simulink model "ctrl_TAPM_2016"  (R2016a)
settings: Solver=ode3  StartTime=0.0  StopTime=inf  FixedStep=0.01  RelTol=1e-3
undefined symbols (not defined in the file): C, D, DiscIntNeverNeededParam, eps_c, epsilon, hd, hd2, I_s, k_cc, K_omega, K_q1f, K_q1r, K_q2f, K_q2r, K_q3f, K_q3r, K_q4f, K_q4r, K_q5f, K_q5r, K_q6f, K_q6r, K_T1f, K_T1r, K_T2f, K_T2r, K_T3f, K_T3r, K_T4f, K_T4r, K_T5f, K_T5r, K_T6f, K_T6r, Kp, Max_Acceleration, Max_rotation, Max_thrust, Min_thrust, n_c, n_max, p_cc, pwm_thr1_backward, pwm_thr1_forward, pwm_thr2_backward, pwm_thr2_forward, pwm_thr3_backward, pwm_thr3_forward, pwm_thr4_backward, pwm_thr4_forward, pwm_thr5_backward, pwm_thr5_forward, pwm_thr6_backward, pwm_thr6_forward, Q_f0, Q_max, r_cc, Rho, Thruster
libraries: marine_gnc x10, dspstat3 x8, simulink x7, simulink_extras x3
(part 4 of 7)

== system ctrl_TAPM_2016/Thruster control  ==
  "Desired thrust and angle " : Inport
  Delay : Delay  DelayLength=1  InitialCondition=0
  Demux : Demux  Outputs=12
  Mapping shaft speed and thrust : Selector  InputPortWidth=12  IndexOptions=Index vector (dialog)  Indices="[1 7 2  8 3 9 4 10 5 11 6 12]"  OutputSizes=1
  Mux : Mux  Inputs=12
  Mux1 : Mux  Inputs=2
  Selecting Desired thrust1 : Selector  InputPortWidth=12  IndexOptions=Index vector (dialog)  Indices=[7 8 9 10 11 12]  OutputSizes=1
  Selecting actual angle : Selector  InputPortWidth=12  IndexOptions=Index vector (dialog)  Indices=[1 2 3 4 5 6]  OutputSizes=1
  Subsystem1 : Subsystem
  Thrust and Shaft speed mapped to PWM : Subsystem
  Thruster 1 : Subsystem
      settings: AttributesFormatString=%<MinAlgLoopOccurrences>
  Thruster 2 : Subsystem
      settings: AttributesFormatString=%<MinAlgLoopOccurrences>
  Thruster 3 : Subsystem
      settings: AttributesFormatString=%<MinAlgLoopOccurrences>
  Thruster 4 : Subsystem
      settings: AttributesFormatString=%<MinAlgLoopOccurrences>
  Thruster 5 : Subsystem
      settings: AttributesFormatString=%<MinAlgLoopOccurrences>
  Thruster 6 : Subsystem
      settings: AttributesFormatString=%<MinAlgLoopOccurrences>
  "Commanded pwm " : Outport
  Commanded angle : Outport  Port=2
  Commanded thrust : Outport  Port=3
  wires:
  Selecting actual angle/1 -> Subsystem1/1(Calculated angles)
  "Desired thrust and angle "/1 -> Selecting actual angle/1, Selecting Desired thrust1/1
  Subsystem1/1(Commanded angles) -> Commanded angle/1
  Thrust and Shaft speed mapped to PWM/1(pwm) -> "Commanded pwm "/1
  Thrust and Shaft speed mapped to PWM/2(Force) -> Commanded thrust/1
  Thrust and Shaft speed mapped to PWM/3("Shaft speed ") -> Delay/1
  Thruster 1/1("Commanded thrust ") -> Mux/1
  Mux/1 -> Thrust and Shaft speed mapped to PWM/1(Calculated thrust)
  Mux1/1 -> Mapping shaft speed and thrust/1
  Delay/1 -> Mux1/2
  Mapping shaft speed and thrust/1 -> Demux/1
  Thruster 1/2(Shaft speed) -> Mux/2
  Demux/2 -> Thruster 1/2(shaft speed)
  Demux/1 -> Thruster 1/1(Desired thrust 1)
  Thruster 2/1("Commanded thrust ") -> Mux/3
  Demux/3 -> Thruster 2/1(Desired thrust 1)
  Demux/4 -> Thruster 2/2(shaft speed)
  Demux/5 -> Thruster 3/1(Desired thrust 1)
  Demux/6 -> Thruster 3/2(shaft speed)
  Demux/7 -> Thruster 4/1(Desired thrust 1)
  Demux/8 -> Thruster 4/2(shaft speed)
  Demux/9 -> Thruster 5/1(Desired thrust 1)
  Demux/10 -> Thruster 5/2(shaft speed)
  Demux/11 -> Thruster 6/1(Desired thrust 1)
  Demux/12 -> Thruster 6/2(shaft speed)
  Thruster 2/2(Shaft speed) -> Mux/4
  Thruster 3/1("Commanded thrust ") -> Mux/5
  Thruster 3/2(Shaft speed) -> Mux/6
  Thruster 4/1("Commanded thrust ") -> Mux/7
  Thruster 4/2(Shaft speed) -> Mux/8
  Thruster 5/1("Commanded thrust ") -> Mux/9
  Thruster 5/2(Shaft speed) -> Mux/10
  Thruster 6/1("Commanded thrust ") -> Mux/11
  Thruster 6/2(Shaft speed) -> Mux/12
  Selecting Desired thrust1/1 -> Mux1/1

== system ctrl_TAPM_2016/Thruster measurment ==
  Mux1 : Mux  Inputs=6
  thr_angle_1 : S-Function  Priority=1  FunctionName=NIVeriStandIO  Parameters=width dtype portnum stime stype btype  SFunctionDeploymentMode=off  EnableBusSupport=off  mask(NI VeriStand Inport){portnum=1, width=-1, stime=-1, dtype=auto, stype=auto, btype=1}
      mask prompts: portnum "Port number:"; width "Port dimensions (-1 for dynamically sized):"; stime "Sample time (-1 for inherited):"; dtype "Data type:"; stype "Signal type:"; btype "Block type:"
      mask help: Use this inport on any level of nested subsystems to allow NI VeriStand software to map signals to it.
      mask init:
      | NIVeriStandIO_init;
      settings: CopyFcn=NIVeriStand_MDL_functions('', 'IO_copy');  DeleteFcn=NIVeriStand_MDL_functions('', 'IO_delete');  MoveFcn=set_param(gcb, 'Mask', 'on');
      mask Callback portnum: NIVeriStand_MDL_functions('', 'IO_setportnum');
      mask TypeOptions dtype: auto | double | single | int8 | uint8 | int16 | uint16 | int32 | uint32 | boolean
      mask Callback dtype: NIVeriStand_MDL_functions('', 'IO_booleansignal');
      mask TypeOptions stype: auto | real | complex
      mask Display:
      | patch([-x x], [-y y], [.90980 .81960 .32156]);
      | plot([xrad -x x xrad], [yrad -y y yrad]);
      | fprintf('NI In%d', portnum);
  thr_angle_2 : S-Function  Priority=2  FunctionName=NIVeriStandIO  Parameters=width dtype portnum stime stype btype  SFunctionDeploymentMode=off  EnableBusSupport=off  mask(NI VeriStand Inport){portnum=2, width=-1, stime=-1, dtype=auto, stype=auto, btype=1}
      mask prompts: portnum "Port number:"; width "Port dimensions (-1 for dynamically sized):"; stime "Sample time (-1 for inherited):"; dtype "Data type:"; stype "Signal type:"; btype "Block type:"
      mask help: Use this inport on any level of nested subsystems to allow NI VeriStand software to map signals to it.
      mask init:
      | NIVeriStandIO_init;
      settings: CopyFcn=NIVeriStand_MDL_functions('', 'IO_copy');  DeleteFcn=NIVeriStand_MDL_functions('', 'IO_delete');  MoveFcn=set_param(gcb, 'Mask', 'on');
      mask Callback portnum: NIVeriStand_MDL_functions('', 'IO_setportnum');
      mask TypeOptions dtype: auto | double | single | int8 | uint8 | int16 | uint16 | int32 | uint32 | boolean
      mask Callback dtype: NIVeriStand_MDL_functions('', 'IO_booleansignal');
      mask TypeOptions stype: auto | real | complex
      mask Display:
      | patch([-x x], [-y y], [.90980 .81960 .32156]);
      | plot([xrad -x x xrad], [yrad -y y yrad]);
      | fprintf('NI In%d', portnum);
  thr_angle_3 : S-Function  Priority=3  FunctionName=NIVeriStandIO  Parameters=width dtype portnum stime stype btype  SFunctionDeploymentMode=off  EnableBusSupport=off  mask(NI VeriStand Inport){portnum=3, width=-1, stime=-1, dtype=auto, stype=auto, btype=1}
      mask prompts: portnum "Port number:"; width "Port dimensions (-1 for dynamically sized):"; stime "Sample time (-1 for inherited):"; dtype "Data type:"; stype "Signal type:"; btype "Block type:"
      mask help: Use this inport on any level of nested subsystems to allow NI VeriStand software to map signals to it.
      mask init:
      | NIVeriStandIO_init;
      settings: CopyFcn=NIVeriStand_MDL_functions('', 'IO_copy');  DeleteFcn=NIVeriStand_MDL_functions('', 'IO_delete');  MoveFcn=set_param(gcb, 'Mask', 'on');
      mask Callback portnum: NIVeriStand_MDL_functions('', 'IO_setportnum');
      mask TypeOptions dtype: auto | double | single | int8 | uint8 | int16 | uint16 | int32 | uint32 | boolean
      mask Callback dtype: NIVeriStand_MDL_functions('', 'IO_booleansignal');
      mask TypeOptions stype: auto | real | complex
      mask Display:
      | patch([-x x], [-y y], [.90980 .81960 .32156]);
      | plot([xrad -x x xrad], [yrad -y y yrad]);
      | fprintf('NI In%d', portnum);
  thr_angle_4 : S-Function  Priority=4  FunctionName=NIVeriStandIO  Parameters=width dtype portnum stime stype btype  SFunctionDeploymentMode=off  EnableBusSupport=off  mask(NI VeriStand Inport){portnum=4, width=-1, stime=-1, dtype=auto, stype=auto, btype=1}
      mask prompts: portnum "Port number:"; width "Port dimensions (-1 for dynamically sized):"; stime "Sample time (-1 for inherited):"; dtype "Data type:"; stype "Signal type:"; btype "Block type:"
      mask help: Use this inport on any level of nested subsystems to allow NI VeriStand software to map signals to it.
      mask init:
      | NIVeriStandIO_init;
      settings: CopyFcn=NIVeriStand_MDL_functions('', 'IO_copy');  DeleteFcn=NIVeriStand_MDL_functions('', 'IO_delete');  MoveFcn=set_param(gcb, 'Mask', 'on');
      mask Callback portnum: NIVeriStand_MDL_functions('', 'IO_setportnum');
      mask TypeOptions dtype: auto | double | single | int8 | uint8 | int16 | uint16 | int32 | uint32 | boolean
      mask Callback dtype: NIVeriStand_MDL_functions('', 'IO_booleansignal');
      mask TypeOptions stype: auto | real | complex
      mask Display:
      | patch([-x x], [-y y], [.90980 .81960 .32156]);
      | plot([xrad -x x xrad], [yrad -y y yrad]);
      | fprintf('NI In%d', portnum);
  thr_angle_5 : S-Function  Priority=5  FunctionName=NIVeriStandIO  Parameters=width dtype portnum stime stype btype  SFunctionDeploymentMode=off  EnableBusSupport=off  mask(NI VeriStand Inport){portnum=5, width=-1, stime=-1, dtype=auto, stype=auto, btype=1}
      mask prompts: portnum "Port number:"; width "Port dimensions (-1 for dynamically sized):"; stime "Sample time (-1 for inherited):"; dtype "Data type:"; stype "Signal type:"; btype "Block type:"
      mask help: Use this inport on any level of nested subsystems to allow NI VeriStand software to map signals to it.
      mask init:
      | NIVeriStandIO_init;
      settings: CopyFcn=NIVeriStand_MDL_functions('', 'IO_copy');  DeleteFcn=NIVeriStand_MDL_functions('', 'IO_delete');  MoveFcn=set_param(gcb, 'Mask', 'on');
      mask Callback portnum: NIVeriStand_MDL_functions('', 'IO_setportnum');
      mask TypeOptions dtype: auto | double | single | int8 | uint8 | int16 | uint16 | int32 | uint32 | boolean
      mask Callback dtype: NIVeriStand_MDL_functions('', 'IO_booleansignal');
      mask TypeOptions stype: auto | real | complex
      mask Display:
      | patch([-x x], [-y y], [.90980 .81960 .32156]);
      | plot([xrad -x x xrad], [yrad -y y yrad]);
      | fprintf('NI In%d', portnum);
  thr_angle_6 : S-Function  Priority=6  FunctionName=NIVeriStandIO  Parameters=width dtype portnum stime stype btype  SFunctionDeploymentMode=off  EnableBusSupport=off  mask(NI VeriStand Inport){portnum=6, width=-1, stime=-1, dtype=auto, stype=auto, btype=1}
      mask prompts: portnum "Port number:"; width "Port dimensions (-1 for dynamically sized):"; stime "Sample time (-1 for inherited):"; dtype "Data type:"; stype "Signal type:"; btype "Block type:"
      mask help: Use this inport on any level of nested subsystems to allow NI VeriStand software to map signals to it.
      mask init:
      | NIVeriStandIO_init;
      settings: CopyFcn=NIVeriStand_MDL_functions('', 'IO_copy');  DeleteFcn=NIVeriStand_MDL_functions('', 'IO_delete');  MoveFcn=set_param(gcb, 'Mask', 'on');
      mask Callback portnum: NIVeriStand_MDL_functions('', 'IO_setportnum');
      mask TypeOptions dtype: auto | double | single | int8 | uint8 | int16 | uint16 | int32 | uint32 | boolean
      mask Callback dtype: NIVeriStand_MDL_functions('', 'IO_booleansignal');
      mask TypeOptions stype: auto | real | complex
      mask Display:
      | patch([-x x], [-y y], [.90980 .81960 .32156]);
      | plot([xrad -x x xrad], [yrad -y y yrad]);
      | fprintf('NI In%d', portnum);
  alpha_m : Outport
  wires:
  thr_angle_3/1 -> Mux1/3
  thr_angle_1/1 -> Mux1/1
  Mux1/1 -> alpha_m/1
  thr_angle_5/1 -> Mux1/5
  thr_angle_4/1 -> Mux1/4
  thr_angle_6/1 -> Mux1/6
  thr_angle_2/1 -> Mux1/2

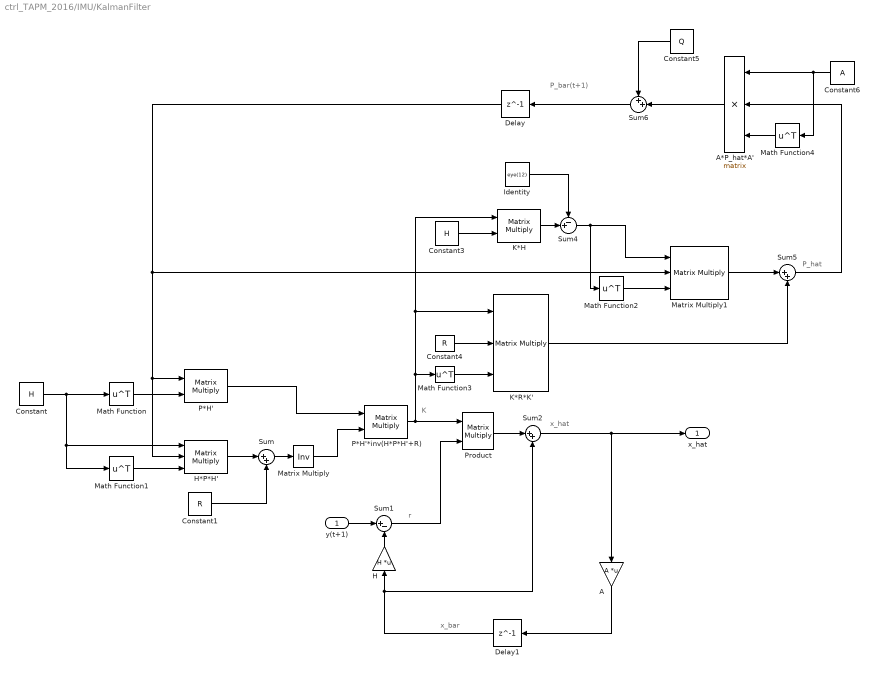
== system ctrl_TAPM_2016/IMU/KalmanFilter ==
  note: P_bar(t+1)
  note: P_hat
  note: x_hat
  note: x_bar
  note: r
  note: K
  y(t+1) : Inport
  A : Gain  Gain=A  Multiplication=Matrix(K*u)
  A*P_hat*A' : Product  Inputs=3  Multiplication=Matrix(*)
  Constant : Constant  Value=H
  Constant1 : Constant  Value=R
  Constant3 : Constant  Value=H
  Constant4 : Constant  Value=R
  Constant5 : Constant  Value=Q
  Constant6 : Constant  Value=A
  Delay : Delay  DelayLength=1  InitialCondition=eye(12)
  Delay1 : Delay  DelayLength=1  InitialCondition=[0 0 0 0 0 0 0 0 0 0 0 0]
  H : Gain  Gain=H  Multiplication=Matrix(K*u)
  H*P*H' : Product  Inputs=3  Multiplication=Matrix(*)
  Identity : Constant  Value=eye(12)
  K*H : Product  Multiplication=Matrix(*)
  K*R*K' : Product  Inputs=3  Multiplication=Matrix(*)
  Math Function{,1..4} (5 alike) : Math  Operator=transpose  SaturateOnIntegerOverflow=on
  Matrix Multiply : Product  Inputs=/  Multiplication=Matrix(*)
  Matrix Multiply1 : Product  Inputs=3  Multiplication=Matrix(*)
  P*H' : Product  Multiplication=Matrix(*)
  P*H'*inv(H*P*H'+R) : Product  Multiplication=Matrix(*)
  Product : Product  Multiplication=Matrix(*)
  Sum : Sum  Inputs=|++
  Sum1 : Sum  Inputs=|+-
  Sum2 : Sum  Inputs=|++
  Sum4 : Sum  Inputs=-+|
  Sum5 : Sum  Inputs=|++
  Sum6 : Sum  Inputs=++|
  x_hat : Outport
  wires:
  Constant/1 -> Math Function1/1, H*P*H'/1, Math Function/1
  Math Function/1 -> P*H'/2
  Math Function1/1 -> H*P*H'/3
  H*P*H'/1 -> Sum/1
  Constant1/1 -> Sum/2
  Sum/1 -> Matrix Multiply/1
  Matrix Multiply/1 -> P*H'*inv(H*P*H'+R)/2
  P*H'/1 -> P*H'*inv(H*P*H'+R)/1
  y(t+1)/1 -> Sum1/1
  H/1 -> Sum1/2
  Delay1/1 -> Sum2/2, H/1
  Sum1/1 -> Product/2
  P*H'*inv(H*P*H'+R)/1 -> K*H/1, K*R*K'/1, Math Function3/1, Product/1
  Product/1 -> Sum2/1
  Sum2/1 -> A/1, x_hat/1
  A/1 -> Delay1/1
  Identity/1 -> Sum4/1
  K*H/1 -> Sum4/2
  Constant3/1 -> K*H/2
  Sum4/1 -> Math Function2/1, Matrix Multiply1/1
  Math Function2/1 -> Matrix Multiply1/3
  Constant4/1 -> K*R*K'/2
  Math Function3/1 -> K*R*K'/3
  K*R*K'/1 -> Sum5/2
  Matrix Multiply1/1 -> Sum5/1
  Sum5/1 -> A*P_hat*A'/2
  Sum6/1 -> Delay/1
  Constant5/1 -> Sum6/1
  A*P_hat*A'/1 -> Sum6/2
  Constant6/1 -> Math Function4/1, A*P_hat*A'/1
  Math Function4/1 -> A*P_hat*A'/3
  Delay/1 -> H*P*H'/2, P*H'/1, Matrix Multiply1/2

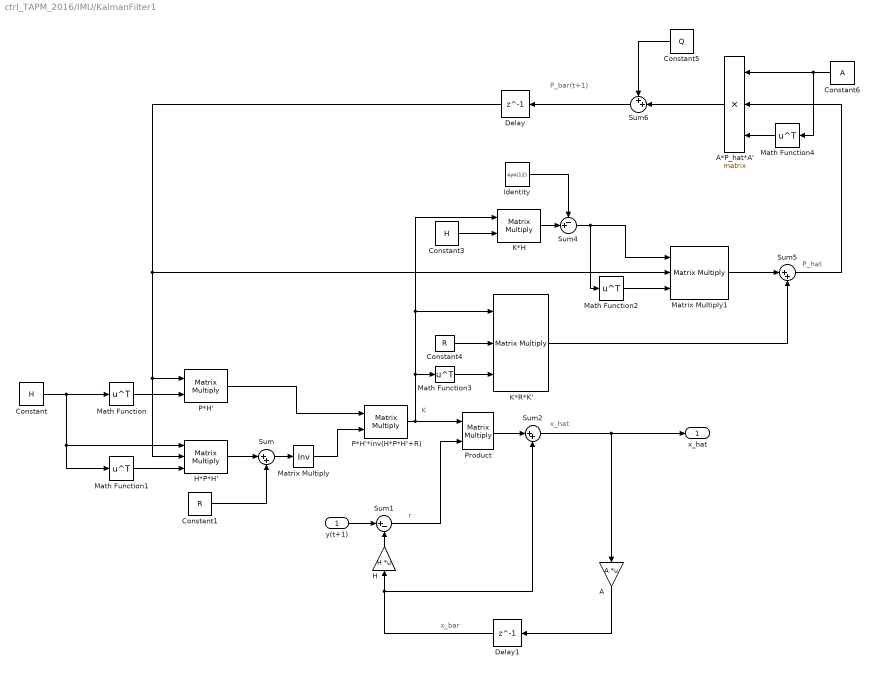
== system ctrl_TAPM_2016/IMU/KalmanFilter1 ==
  note: P_bar(t+1)
  note: P_hat
  note: x_hat
  note: x_bar
  note: r
  note: K
  y(t+1) : Inport
  A : Gain  Gain=A  Multiplication=Matrix(K*u)
  A*P_hat*A' : Product  Inputs=3  Multiplication=Matrix(*)
  Constant : Constant  Value=H
  Constant1 : Constant  Value=R
  Constant3 : Constant  Value=H
  Constant4 : Constant  Value=R
  Constant5 : Constant  Value=Q
  Constant6 : Constant  Value=A
  Delay : Delay  DelayLength=1  InitialCondition=eye(12)
  Delay1 : Delay  DelayLength=1  InitialCondition=[0 0 0 0 0 0 0 0 0 0 0 0]
  H : Gain  Gain=H  Multiplication=Matrix(K*u)
  H*P*H' : Product  Inputs=3  Multiplication=Matrix(*)
  Identity : Constant  Value=eye(12)
  K*H : Product  Multiplication=Matrix(*)
  K*R*K' : Product  Inputs=3  Multiplication=Matrix(*)
  Math Function{,1..4} (5 alike) : Math  Operator=transpose  SaturateOnIntegerOverflow=on
  Matrix Multiply : Product  Inputs=/  Multiplication=Matrix(*)
  Matrix Multiply1 : Product  Inputs=3  Multiplication=Matrix(*)
  P*H' : Product  Multiplication=Matrix(*)
  P*H'*inv(H*P*H'+R) : Product  Multiplication=Matrix(*)
  Product : Product  Multiplication=Matrix(*)
  Sum : Sum  Inputs=|++
  Sum1 : Sum  Inputs=|+-
  Sum2 : Sum  Inputs=|++
  Sum4 : Sum  Inputs=-+|
  Sum5 : Sum  Inputs=|++
  Sum6 : Sum  Inputs=++|
  x_hat : Outport
  wires:
  Constant/1 -> Math Function1/1, H*P*H'/1, Math Function/1
  Math Function/1 -> P*H'/2
  Math Function1/1 -> H*P*H'/3
  H*P*H'/1 -> Sum/1
  Constant1/1 -> Sum/2
  Sum/1 -> Matrix Multiply/1
  Matrix Multiply/1 -> P*H'*inv(H*P*H'+R)/2
  P*H'/1 -> P*H'*inv(H*P*H'+R)/1
  y(t+1)/1 -> Sum1/1
  H/1 -> Sum1/2
  Delay1/1 -> Sum2/2, H/1
  Sum1/1 -> Product/2
  P*H'*inv(H*P*H'+R)/1 -> K*H/1, K*R*K'/1, Math Function3/1, Product/1
  Product/1 -> Sum2/1
  Sum2/1 -> A/1, x_hat/1
  A/1 -> Delay1/1
  Identity/1 -> Sum4/1
  K*H/1 -> Sum4/2
  Constant3/1 -> K*H/2
  Sum4/1 -> Math Function2/1, Matrix Multiply1/1
  Math Function2/1 -> Matrix Multiply1/3
  Constant4/1 -> K*R*K'/2
  Math Function3/1 -> K*R*K'/3
  K*R*K'/1 -> Sum5/2
  Matrix Multiply1/1 -> Sum5/1
  Sum5/1 -> A*P_hat*A'/2
  Sum6/1 -> Delay/1
  Constant5/1 -> Sum6/1
  A*P_hat*A'/1 -> Sum6/2
  Constant6/1 -> Math Function4/1, A*P_hat*A'/1
  Math Function4/1 -> A*P_hat*A'/3
  Delay/1 -> H*P*H'/2, P*H'/1, Matrix Multiply1/2

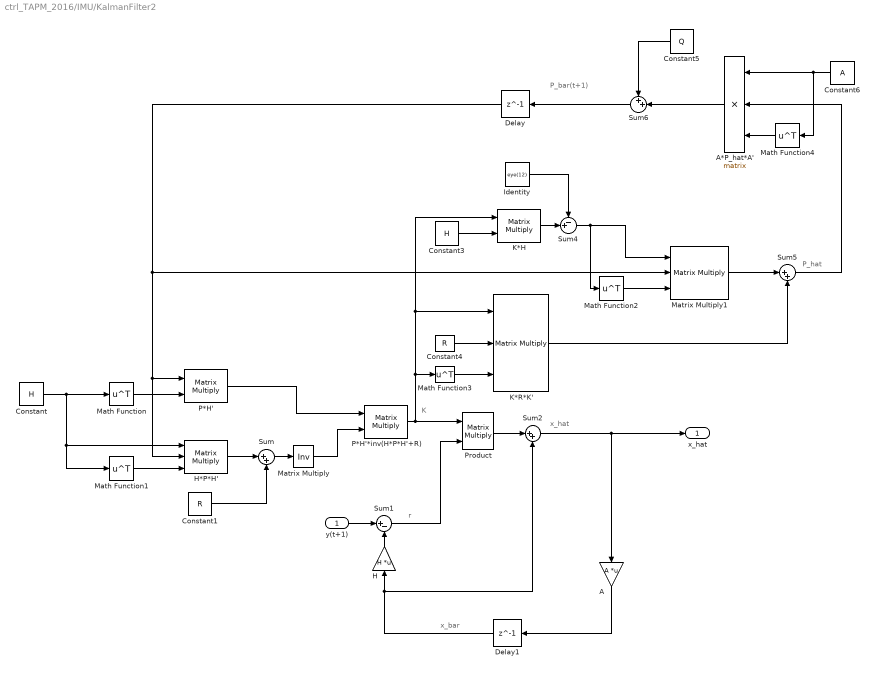
== system ctrl_TAPM_2016/IMU/KalmanFilter2 ==
  note: P_bar(t+1)
  note: P_hat
  note: x_hat
  note: x_bar
  note: r
  note: K
  y(t+1) : Inport
  A : Gain  Gain=A  Multiplication=Matrix(K*u)
  A*P_hat*A' : Product  Inputs=3  Multiplication=Matrix(*)
  Constant : Constant  Value=H
  Constant1 : Constant  Value=R
  Constant3 : Constant  Value=H
  Constant4 : Constant  Value=R
  Constant5 : Constant  Value=Q
  Constant6 : Constant  Value=A
  Delay : Delay  DelayLength=1  InitialCondition=eye(12)
  Delay1 : Delay  DelayLength=1  InitialCondition=[0 0 0 0 0 0 0 0 0 0 0 0]
  H : Gain  Gain=H  Multiplication=Matrix(K*u)
  H*P*H' : Product  Inputs=3  Multiplication=Matrix(*)
  Identity : Constant  Value=eye(12)
  K*H : Product  Multiplication=Matrix(*)
  K*R*K' : Product  Inputs=3  Multiplication=Matrix(*)
  Math Function{,1..4} (5 alike) : Math  Operator=transpose  SaturateOnIntegerOverflow=on
  Matrix Multiply : Product  Inputs=/  Multiplication=Matrix(*)
  Matrix Multiply1 : Product  Inputs=3  Multiplication=Matrix(*)
  P*H' : Product  Multiplication=Matrix(*)
  P*H'*inv(H*P*H'+R) : Product  Multiplication=Matrix(*)
  Product : Product  Multiplication=Matrix(*)
  Sum : Sum  Inputs=|++
  Sum1 : Sum  Inputs=|+-
  Sum2 : Sum  Inputs=|++
  Sum4 : Sum  Inputs=-+|
  Sum5 : Sum  Inputs=|++
  Sum6 : Sum  Inputs=++|
  x_hat : Outport
  wires:
  Constant/1 -> Math Function1/1, H*P*H'/1, Math Function/1
  Math Function/1 -> P*H'/2
  Math Function1/1 -> H*P*H'/3
  H*P*H'/1 -> Sum/1
  Constant1/1 -> Sum/2
  Sum/1 -> Matrix Multiply/1
  Matrix Multiply/1 -> P*H'*inv(H*P*H'+R)/2
  P*H'/1 -> P*H'*inv(H*P*H'+R)/1
  y(t+1)/1 -> Sum1/1
  H/1 -> Sum1/2
  Delay1/1 -> Sum2/2, H/1
  Sum1/1 -> Product/2
  P*H'*inv(H*P*H'+R)/1 -> K*H/1, K*R*K'/1, Math Function3/1, Product/1
  Product/1 -> Sum2/1
  Sum2/1 -> A/1, x_hat/1
  A/1 -> Delay1/1
  Identity/1 -> Sum4/1
  K*H/1 -> Sum4/2
  Constant3/1 -> K*H/2
  Sum4/1 -> Math Function2/1, Matrix Multiply1/1
  Math Function2/1 -> Matrix Multiply1/3
  Constant4/1 -> K*R*K'/2
  Math Function3/1 -> K*R*K'/3
  K*R*K'/1 -> Sum5/2
  Matrix Multiply1/1 -> Sum5/1
  Sum5/1 -> A*P_hat*A'/2
  Sum6/1 -> Delay/1
  Constant5/1 -> Sum6/1
  A*P_hat*A'/1 -> Sum6/2
  Constant6/1 -> Math Function4/1, A*P_hat*A'/1
  Math Function4/1 -> A*P_hat*A'/3
  Delay/1 -> H*P*H'/2, P*H'/1, Matrix Multiply1/2

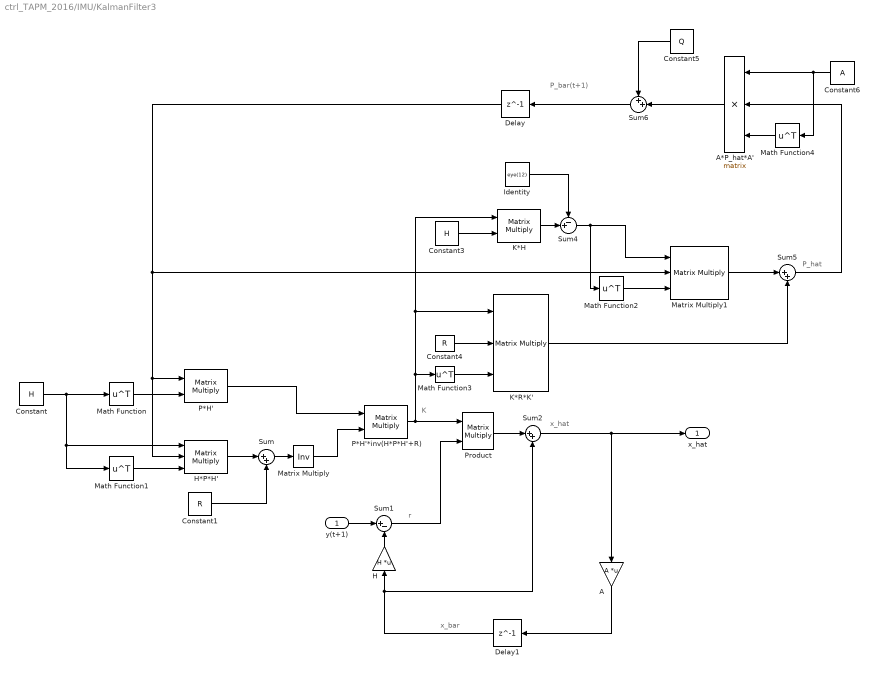
== system ctrl_TAPM_2016/IMU/KalmanFilter3 ==
  note: P_bar(t+1)
  note: P_hat
  note: x_hat
  note: x_bar
  note: r
  note: K
  y(t+1) : Inport
  A : Gain  Gain=A  Multiplication=Matrix(K*u)
  A*P_hat*A' : Product  Inputs=3  Multiplication=Matrix(*)
  Constant : Constant  Value=H
  Constant1 : Constant  Value=R
  Constant3 : Constant  Value=H
  Constant4 : Constant  Value=R
  Constant5 : Constant  Value=Q
  Constant6 : Constant  Value=A
  Delay : Delay  DelayLength=1  InitialCondition=eye(12)
  Delay1 : Delay  DelayLength=1  InitialCondition=[0 0 0 0 0 0 0 0 0 0 0 0]
  H : Gain  Gain=H  Multiplication=Matrix(K*u)
  H*P*H' : Product  Inputs=3  Multiplication=Matrix(*)
  Identity : Constant  Value=eye(12)
  K*H : Product  Multiplication=Matrix(*)
  K*R*K' : Product  Inputs=3  Multiplication=Matrix(*)
  Math Function{,1..4} (5 alike) : Math  Operator=transpose  SaturateOnIntegerOverflow=on
  Matrix Multiply : Product  Inputs=/  Multiplication=Matrix(*)
  Matrix Multiply1 : Product  Inputs=3  Multiplication=Matrix(*)
  P*H' : Product  Multiplication=Matrix(*)
  P*H'*inv(H*P*H'+R) : Product  Multiplication=Matrix(*)
  Product : Product  Multiplication=Matrix(*)
  Sum : Sum  Inputs=|++
  Sum1 : Sum  Inputs=|+-
  Sum2 : Sum  Inputs=|++
  Sum4 : Sum  Inputs=-+|
  Sum5 : Sum  Inputs=|++
  Sum6 : Sum  Inputs=++|
  x_hat : Outport
  wires:
  Constant/1 -> Math Function1/1, H*P*H'/1, Math Function/1
  Math Function/1 -> P*H'/2
  Math Function1/1 -> H*P*H'/3
  H*P*H'/1 -> Sum/1
  Constant1/1 -> Sum/2
  Sum/1 -> Matrix Multiply/1
  Matrix Multiply/1 -> P*H'*inv(H*P*H'+R)/2
  P*H'/1 -> P*H'*inv(H*P*H'+R)/1
  y(t+1)/1 -> Sum1/1
  H/1 -> Sum1/2
  Delay1/1 -> Sum2/2, H/1
  Sum1/1 -> Product/2
  P*H'*inv(H*P*H'+R)/1 -> K*H/1, K*R*K'/1, Math Function3/1, Product/1
  Product/1 -> Sum2/1
  Sum2/1 -> A/1, x_hat/1
  A/1 -> Delay1/1
  Identity/1 -> Sum4/1
  K*H/1 -> Sum4/2
  Constant3/1 -> K*H/2
  Sum4/1 -> Math Function2/1, Matrix Multiply1/1
  Math Function2/1 -> Matrix Multiply1/3
  Constant4/1 -> K*R*K'/2
  Math Function3/1 -> K*R*K'/3
  K*R*K'/1 -> Sum5/2
  Matrix Multiply1/1 -> Sum5/1
  Sum5/1 -> A*P_hat*A'/2
  Sum6/1 -> Delay/1
  Constant5/1 -> Sum6/1
  A*P_hat*A'/1 -> Sum6/2
  Constant6/1 -> Math Function4/1, A*P_hat*A'/1
  Math Function4/1 -> A*P_hat*A'/3
  Delay/1 -> H*P*H'/2, P*H'/1, Matrix Multiply1/2

== system ctrl_TAPM_2016/IMU/Outliner cleaner ==
  Y : Inport
  Abs : Abs
  Abs1 : Abs
  Gain : Gain  Gain=2*1.4826
  If : If  NumInputs=2  IfExpression=u1 < u2
  Median : dspstat3/Median  sortAlg=Quick sort  directionMode=Entire input  dimension=1  outputDataTypeStr=Inherit: Same as accumulator  outputLastDataTypeStr=Inherit: Same as accumulator  outputMin=[]  outputMax=[]  accumDataTypeStr=Inherit: Same as product output  accumLastDataTypeStr=Inherit: Same as product output  roundingMode=Floor  overflowMode=off
      settings: allowOverrides=off
  Median1 : dspstat3/Median  sortAlg=Quick sort  directionMode=Entire input  dimension=1  outputDataTypeStr=Inherit: Same as accumulator  outputLastDataTypeStr=Inherit: Same as accumulator  outputMin=[]  outputMax=[]  accumDataTypeStr=Inherit: Same as product output  accumLastDataTypeStr=Inherit: Same as product output  roundingMode=Floor  overflowMode=off
      settings: allowOverrides=off
  Memory2 : Memory  X0=[4.968, 4.965, 4.97, 4.975, 4.96]
  Memory3 : Memory  X0=[0, 0, 0, 0, 0, 0, 0]
  Merge : Merge
  Merge1 : Merge
  No outlier : Subsystem  TreatAsAtomicUnit=on
  Outlier detected : Subsystem  TreatAsAtomicUnit=on
  Selector : Selector  InputPortWidth=7  IndexOptions=Index vector (dialog)  Indices=[7]  OutputSizes=1
  Sum : Sum  Inputs=+-|
  Sum1 : Sum  Inputs=-+|
  Y2 : InportShadow
  Y_filtered : Outport
  wires:
  Memory2/1 -> Sum/1, [V_old], Median/1
  Median/1 -> Sum1/1, Sum/2
  Sum/1 -> Abs/1
  Abs/1 -> Median1/1
  Y/1 -> Memory3/1, Selector/1
  Selector/1 -> Sum1/2
  Sum1/1 -> Abs1/1
  Abs1/1 -> If/2
  Gain/1 -> If/1
  [Y_prev] -> Outlier detected/1(Y_previous)
  Outlier detected/1(Y_filtered) -> Merge/1
  If/1 -> Outlier detected/Action
  If/2 -> No outlier/Action
  Y2/1 -> No outlier/1(Y)
  Merge1/1 -> Memory2/1
  No outlier/1(Y_filtered) -> Merge/2
  Median1/1 -> Gain/1
  Memory3/1 -> [Y_prev]
  Merge/1 -> Y_filtered/1
  [V_old] -> Outlier detected/2(V)
  Outlier detected/2(V_hist) -> Merge1/1
  [V_old] -> No outlier/2(V)
  No outlier/2(V_hist) -> Merge1/2

== system ctrl_TAPM_2016/IMU/Outliner cleaner1 ==
  Y : Inport
  Abs : Abs
  Abs1 : Abs
  Gain : Gain  Gain=2*1.4826
  If : If  NumInputs=2  IfExpression=u1 < u2
  Median : dspstat3/Median  sortAlg=Quick sort  directionMode=Entire input  dimension=1  outputDataTypeStr=Inherit: Same as accumulator  outputLastDataTypeStr=Inherit: Same as accumulator  outputMin=[]  outputMax=[]  accumDataTypeStr=Inherit: Same as product output  accumLastDataTypeStr=Inherit: Same as product output  roundingMode=Floor  overflowMode=off
      settings: allowOverrides=off
  Median1 : dspstat3/Median  sortAlg=Quick sort  directionMode=Entire input  dimension=1  outputDataTypeStr=Inherit: Same as accumulator  outputLastDataTypeStr=Inherit: Same as accumulator  outputMin=[]  outputMax=[]  accumDataTypeStr=Inherit: Same as product output  accumLastDataTypeStr=Inherit: Same as product output  roundingMode=Floor  overflowMode=off
      settings: allowOverrides=off
  Memory2 : Memory  X0=[4.968, 4.965, 4.97, 4.975, 4.96]
  Memory3 : Memory  X0=[0, 0, 0, 0, 0, 0, 0]
  Merge : Merge
  Merge1 : Merge
  No outlier : Subsystem  TreatAsAtomicUnit=on
  Outlier detected : Subsystem  TreatAsAtomicUnit=on
  Selector : Selector  InputPortWidth=7  IndexOptions=Index vector (dialog)  Indices=[7]  OutputSizes=1
  Sum : Sum  Inputs=+-|
  Sum1 : Sum  Inputs=-+|
  Y2 : InportShadow
  Y_filtered : Outport
  wires:
  Memory2/1 -> Sum/1, [V_old], Median/1
  Median/1 -> Sum1/1, Sum/2
  Sum/1 -> Abs/1
  Abs/1 -> Median1/1
  Y/1 -> Memory3/1, Selector/1
  Selector/1 -> Sum1/2
  Sum1/1 -> Abs1/1
  Abs1/1 -> If/2
  Gain/1 -> If/1
  [Y_prev] -> Outlier detected/1(Y_previous)
  Outlier detected/1(Y_filtered) -> Merge/1
  If/1 -> Outlier detected/Action
  If/2 -> No outlier/Action
  Y2/1 -> No outlier/1(Y)
  Merge1/1 -> Memory2/1
  No outlier/1(Y_filtered) -> Merge/2
  Median1/1 -> Gain/1
  Memory3/1 -> [Y_prev]
  Merge/1 -> Y_filtered/1
  [V_old] -> Outlier detected/2(V)
  Outlier detected/2(V_hist) -> Merge1/1
  [V_old] -> No outlier/2(V)
  No outlier/2(V_hist) -> Merge1/2

== system ctrl_TAPM_2016/IMU/Outliner cleaner2 ==
  Y : Inport
  Abs : Abs
  Abs1 : Abs
  Gain : Gain  Gain=2*1.4826
  If : If  NumInputs=2  IfExpression=u1 < u2
  Median : dspstat3/Median  sortAlg=Quick sort  directionMode=Entire input  dimension=1  outputDataTypeStr=Inherit: Same as accumulator  outputLastDataTypeStr=Inherit: Same as accumulator  outputMin=[]  outputMax=[]  accumDataTypeStr=Inherit: Same as product output  accumLastDataTypeStr=Inherit: Same as product output  roundingMode=Floor  overflowMode=off
      settings: allowOverrides=off
  Median1 : dspstat3/Median  sortAlg=Quick sort  directionMode=Entire input  dimension=1  outputDataTypeStr=Inherit: Same as accumulator  outputLastDataTypeStr=Inherit: Same as accumulator  outputMin=[]  outputMax=[]  accumDataTypeStr=Inherit: Same as product output  accumLastDataTypeStr=Inherit: Same as product output  roundingMode=Floor  overflowMode=off
      settings: allowOverrides=off
  Memory2 : Memory  X0=[4.968, 4.965, 4.97, 4.975, 4.96]
  Memory3 : Memory  X0=[0, 0, 0, 0, 0, 0, 0]
  Merge : Merge
  Merge1 : Merge
  No outlier : Subsystem  TreatAsAtomicUnit=on
  Outlier detected : Subsystem  TreatAsAtomicUnit=on
  Selector : Selector  InputPortWidth=7  IndexOptions=Index vector (dialog)  Indices=[7]  OutputSizes=1
  Sum : Sum  Inputs=+-|
  Sum1 : Sum  Inputs=-+|
  Y2 : InportShadow
  Y_filtered : Outport
  wires:
  Memory2/1 -> Sum/1, [V_old], Median/1
  Median/1 -> Sum1/1, Sum/2
  Sum/1 -> Abs/1
  Abs/1 -> Median1/1
  Y/1 -> Memory3/1, Selector/1
  Selector/1 -> Sum1/2
  Sum1/1 -> Abs1/1
  Abs1/1 -> If/2
  Gain/1 -> If/1
  [Y_prev] -> Outlier detected/1(Y_previous)
  Outlier detected/1(Y_filtered) -> Merge/1
  If/1 -> Outlier detected/Action
  If/2 -> No outlier/Action
  Y2/1 -> No outlier/1(Y)
  Merge1/1 -> Memory2/1
  No outlier/1(Y_filtered) -> Merge/2
  Median1/1 -> Gain/1
  Memory3/1 -> [Y_prev]
  Merge/1 -> Y_filtered/1
  [V_old] -> Outlier detected/2(V)
  Outlier detected/2(V_hist) -> Merge1/1
  [V_old] -> No outlier/2(V)
  No outlier/2(V_hist) -> Merge1/2

== system ctrl_TAPM_2016/IMU/Outliner cleaner3 ==
  Y : Inport
  Abs : Abs
  Abs1 : Abs
  Gain : Gain  Gain=2*1.4826
  If : If  NumInputs=2  IfExpression=u1 < u2
  Median : dspstat3/Median  sortAlg=Quick sort  directionMode=Entire input  dimension=1  outputDataTypeStr=Inherit: Same as accumulator  outputLastDataTypeStr=Inherit: Same as accumulator  outputMin=[]  outputMax=[]  accumDataTypeStr=Inherit: Same as product output  accumLastDataTypeStr=Inherit: Same as product output  roundingMode=Floor  overflowMode=off
      settings: allowOverrides=off
  Median1 : dspstat3/Median  sortAlg=Quick sort  directionMode=Entire input  dimension=1  outputDataTypeStr=Inherit: Same as accumulator  outputLastDataTypeStr=Inherit: Same as accumulator  outputMin=[]  outputMax=[]  accumDataTypeStr=Inherit: Same as product output  accumLastDataTypeStr=Inherit: Same as product output  roundingMode=Floor  overflowMode=off
      settings: allowOverrides=off
  Memory2 : Memory  X0=[4.968, 4.965, 4.97, 4.975, 4.96]
  Memory3 : Memory  X0=[0, 0, 0, 0, 0, 0, 0]
  Merge : Merge
  Merge1 : Merge
  No outlier : Subsystem  TreatAsAtomicUnit=on
  Outlier detected : Subsystem  TreatAsAtomicUnit=on
  Selector : Selector  InputPortWidth=7  IndexOptions=Index vector (dialog)  Indices=[7]  OutputSizes=1
  Sum : Sum  Inputs=+-|
  Sum1 : Sum  Inputs=-+|
  Y2 : InportShadow
  Y_filtered : Outport
  wires:
  Memory2/1 -> Sum/1, [V_old], Median/1
  Median/1 -> Sum1/1, Sum/2
  Sum/1 -> Abs/1
  Abs/1 -> Median1/1
  Y/1 -> Memory3/1, Selector/1
  Selector/1 -> Sum1/2
  Sum1/1 -> Abs1/1
  Abs1/1 -> If/2
  Gain/1 -> If/1
  [Y_prev] -> Outlier detected/1(Y_previous)
  Outlier detected/1(Y_filtered) -> Merge/1
  If/1 -> Outlier detected/Action
  If/2 -> No outlier/Action
  Y2/1 -> No outlier/1(Y)
  Merge1/1 -> Memory2/1
  No outlier/1(Y_filtered) -> Merge/2
  Median1/1 -> Gain/1
  Memory3/1 -> [Y_prev]
  Merge/1 -> Y_filtered/1
  [V_old] -> Outlier detected/2(V)
  Outlier detected/2(V_hist) -> Merge1/1
  [V_old] -> No outlier/2(V)
  No outlier/2(V_hist) -> Merge1/2

== system ctrl_TAPM_2016/IMU/Wild point cleaner ==
  Y : Inport
  MATLAB Function : MATLAB Function  Commented=on  TreatAsAtomicUnit=on
  Memory : Memory  Commented=on  X0=[4.968, 4.965, 4.97, 4.975, 4.96]
  Memory1 : Memory  Commented=on  X0=[0, 0, 0, 0, 0, 0, 0]
  wires:
  Y/1 -> MATLAB Function/2(Y)
  MATLAB Function/2(Y_filtered) -> Memory1/1
  MATLAB Function/1(V_hist1) -> Memory/1
  Memory/1 -> MATLAB Function/1(V_hist)
  Memory1/1 -> MATLAB Function/3(Y_prev)

== system ctrl_TAPM_2016/TAPM Controller w_observer/LQR ==
  SP : Inport
  eta : Inport  Port=2
  bias : Inport  Port=3
  Constant : Constant
  Delay : Delay  DelayLength=1  InitialCondition=0
  Integrator : Integrator  ExternalReset=rising  IgnoreLimit=on
  MATLAB Function : MATLAB Function  TreatAsAtomicUnit=on
  MATLAB Function1 : MATLAB Function  TreatAsAtomicUnit=on
  MATLAB Function2 : MATLAB Function  TreatAsAtomicUnit=on
  MATLAB Function3 : MATLAB Function  TreatAsAtomicUnit=on
  Multiport Switch : MultiPortSwitch  Inputs=2
  controller : S-Function  Priority=1  FunctionName=NIVeriStandIO  Parameters=width dtype portnum stime stype btype  SFunctionDeploymentMode=off  EnableBusSupport=off  mask(NI VeriStand Outport){portnum=1, width=-1, stime=-1, dtype=auto, stype=auto, btype=0}
      mask prompts: portnum "Port number:"; width "Port dimensions (-1 for dynamically sized):"; stime "Sample time (-1 for inherited):"; dtype "Data type:"; stype "Signal type:"; btype "Block type:"
      mask help: Use this outport on any level of nested subsystems to allow NI VeriStand software to map signals to it.
      mask init:
      | NIVeriStandIO_init;
      settings: CopyFcn=NIVeriStand_MDL_functions('', 'IO_copy');  DeleteFcn=NIVeriStand_MDL_functions('', 'IO_delete');  MoveFcn=set_param(gcb, 'Mask', 'on');
      mask Callback portnum: NIVeriStand_MDL_functions('', 'IO_setportnum');
      mask TypeOptions dtype: auto | double | single | int8 | uint8 | int16 | uint16 | int32 | uint32 | boolean
      mask Callback dtype: NIVeriStand_MDL_functions('', 'IO_booleansignal');
      mask TypeOptions stype: auto | real | complex
      mask Display:
      | patch([-x x], [-y y], [.90980 .81960 .32156]);
      | plot([xrad -x x xrad], [yrad -y y yrad]);
      | fprintf('NI Out%d', portnum);
  timer : S-Function  Priority=2  FunctionName=NIVeriStandIO  Parameters=width dtype portnum stime stype btype  SFunctionDeploymentMode=off  EnableBusSupport=off  mask(NI VeriStand Outport){portnum=2, width=-1, stime=-1, dtype=auto, stype=auto, btype=0}
      mask prompts: portnum "Port number:"; width "Port dimensions (-1 for dynamically sized):"; stime "Sample time (-1 for inherited):"; dtype "Data type:"; stype "Signal type:"; btype "Block type:"
      mask help: Use this outport on any level of nested subsystems to allow NI VeriStand software to map signals to it.
      mask init:
      | NIVeriStandIO_init;
      settings: CopyFcn=NIVeriStand_MDL_functions('', 'IO_copy');  DeleteFcn=NIVeriStand_MDL_functions('', 'IO_delete');  MoveFcn=set_param(gcb, 'Mask', 'on');
      mask Callback portnum: NIVeriStand_MDL_functions('', 'IO_setportnum');
      mask TypeOptions dtype: auto | double | single | int8 | uint8 | int16 | uint16 | int32 | uint32 | boolean
      mask Callback dtype: NIVeriStand_MDL_functions('', 'IO_booleansignal');
      mask TypeOptions stype: auto | real | complex
      mask Display:
      | patch([-x x], [-y y], [.90980 .81960 .32156]);
      | plot([xrad -x x xrad], [yrad -y y yrad]);
      | fprintf('NI Out%d', portnum);
  tau_d : Outport  PortDimensions=3
  wires:
  SP/1 -> MATLAB Function3/1(r), MATLAB Function1/1(r)
  eta/1 -> MATLAB Function/3(eta), MATLAB Function1/2(x_hat), MATLAB Function3/2(x_hat)
  Constant/1 -> Integrator/1
  MATLAB Function/1(reset) -> Integrator/2
  Integrator/1 -> Delay/1
  MATLAB Function/2(y) -> controller/1, Multiport Switch/1
  Delay/1 -> timer/1, MATLAB Function/1(timer)
  bias/1 -> MATLAB Function1/3(bias), MATLAB Function3/3(bias)
  [r_max] -> MATLAB Function/2(rmax)
  Multiport Switch/1 -> MATLAB Function2/1(u)
  MATLAB Function1/1(tau) -> Multiport Switch/2
  MATLAB Function3/1(tau) -> Multiport Switch/3
  MATLAB Function2/1(y) -> tau_d/1

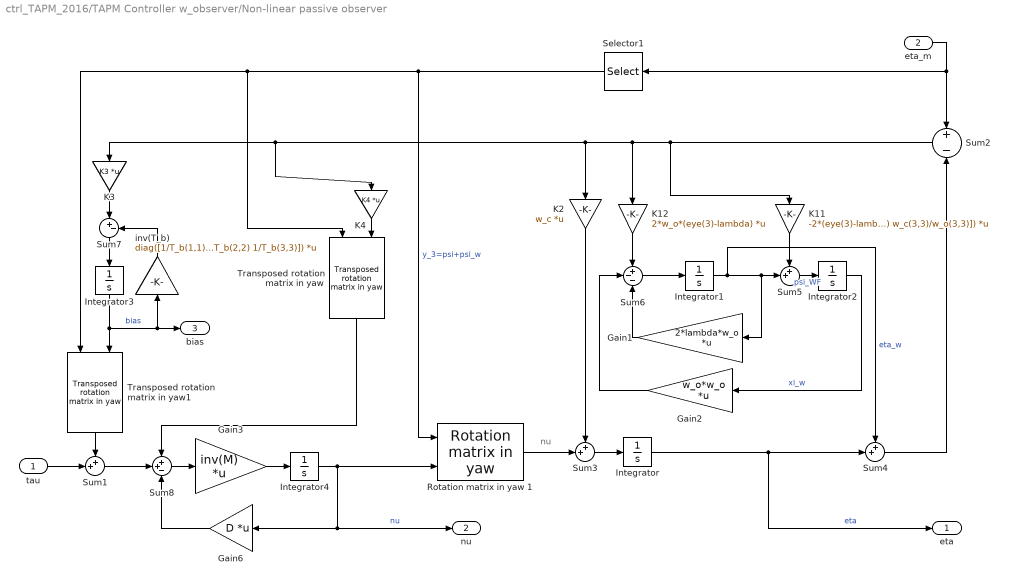
== system ctrl_TAPM_2016/TAPM Controller w_observer/Non-linear passive observer  ==
  note: nu
  tau : Inport
  eta_m : Inport  Port=2
  Gain1 : Gain  Gain=2*lambda*w_o  Multiplication=Matrix(K*u)  SaturateOnIntegerOverflow=on  OutDataTypeStr=Inherit: Same as input  ParamDataTypeStr=Inherit: Same as input
  Gain2 : Gain  Gain=w_o*w_o  Multiplication=Matrix(K*u)  SaturateOnIntegerOverflow=on  OutDataTypeStr=Inherit: Same as input  ParamDataTypeStr=Inherit: Same as input
  Gain3 : Gain  Gain=inv(M)  Multiplication=Matrix(K*u)  SaturateOnIntegerOverflow=on  OutDataTypeStr=Inherit: Same as input  ParamDataTypeStr=Inherit: Same as input
  Gain6 : Gain  Gain=D  Multiplication=Matrix(K*u)  SaturateOnIntegerOverflow=on  OutDataTypeStr=Inherit: Same as input  ParamDataTypeStr=Inherit: Same as input
  Integrator : Integrator  InitialCondition=[0,0,0]'
  Integrator1 : Integrator
  Integrator2 : Integrator
  Integrator3 : Integrator
  Integrator4 : Integrator  InitialCondition=[0,0,0]'
  K11 : Gain  Gain=-2*(eye(3)-lambda)*diag([w_c(1,1)/w_o(1,1) w_c(2,2)/w_o(2,2) w_c(3,3)/w_o(3,3)])  Multiplication=Matrix(K*u)  SaturateOnIntegerOverflow=on  OutDataTypeStr=Inherit: Same as input  ParamDataTypeStr=Inherit: Same as input
  K12 : Gain  Gain=2*w_o*(eye(3)-lambda)  Multiplication=Matrix(K*u)  SaturateOnIntegerOverflow=on  OutDataTypeStr=Inherit: Same as input  ParamDataTypeStr=Inherit: Same as input
  K2 : Gain  Gain=w_c  Multiplication=Matrix(K*u)  SaturateOnIntegerOverflow=on  OutDataTypeStr=Inherit: Same as input  ParamDataTypeStr=Inherit: Same as input
  K3 : Gain  Gain=K3  Multiplication=Matrix(K*u)  SaturateOnIntegerOverflow=on  OutDataTypeStr=Inherit: Same as input  ParamDataTypeStr=Inherit: Same as input
  K4 : Gain  Gain=K4  Multiplication=Matrix(K*u)  SaturateOnIntegerOverflow=on  OutDataTypeStr=Inherit: Same as input  ParamDataTypeStr=Inherit: Same as input
  Rotation matrix in yaw 1 : marine_gnc/Models/ Kinematics/Rotation matrix in yaw 
  Selector1 : Selector  InputPortWidth=3  IndexOptions=Index vector (dialog)  Indices=[3]  OutputSizes=1
  Sum{1,3..5} (4 alike) : Sum  Inputs=++|  SaturateOnIntegerOverflow=on  InputSameDT=on  OutDataTypeStr=Inherit: Same as first input
  Sum2 : Sum  Inputs=+|-  SaturateOnIntegerOverflow=on  InputSameDT=on  OutDataTypeStr=Inherit: Same as first input
  Sum6 : Sum  Inputs=+--  SaturateOnIntegerOverflow=on  InputSameDT=on  OutDataTypeStr=Inherit: Same as first input
  Sum7 : Sum  Inputs=|+-  SaturateOnIntegerOverflow=on  InputSameDT=on  OutDataTypeStr=Inherit: Same as first input
  Sum8 : Sum  Inputs=++-  SaturateOnIntegerOverflow=on  InputSameDT=on  OutDataTypeStr=Inherit: Same as first input
  Transposed rotation matrix in yaw : marine_gnc/Models/ Kinematics/Transposed rotation  matrix in yaw
  Transposed rotation matrix in yaw1 : marine_gnc/Models/ Kinematics/Transposed rotation  matrix in yaw
  inv(T_b) : Gain  Gain=diag([1/T_b(1,1) 1/T_b(2,2) 1/T_b(3,3)])  Multiplication=Matrix(K*u)  SaturateOnIntegerOverflow=on  OutDataTypeStr=Inherit: Same as input  ParamDataTypeStr=Inherit: Same as input
  eta : Outport
  nu : Outport  Port=2
  bias : Outport  Port=3  PortDimensions=3
  wires:
  Sum3/1 -> Integrator/1
  Integrator2/1 -> Gain2/1  "xi_w"
  Gain2/1 -> Sum6/2
  Sum6/1 -> Integrator1/1
  Sum4/1 -> Sum2/2
  Sum2/1 -> K4/1, K3/1, K2/1, K12/1, K11/1
  Gain1/1 -> Sum6/3
  K2/1 -> Sum3/1
  Integrator/1 -> Sum4/2, eta/1  "eta"
  inv(T_b)/1 -> Sum7/2
  Integrator3/1 -> Transposed rotation matrix in yaw1/2, bias/1, inv(T_b)/1  "bias"
  tau/1 -> Sum1/2
  Integrator1/1 -> Sum4/1, Gain1/1, Sum5/2  "eta_w"
  K12/1 -> Sum6/1
  K11/1 -> Sum5/1
  eta_m/1 -> Selector1/1, Sum2/1
  Sum5/1 -> Integrator2/1  "psi_WF"
  Sum7/1 -> Integrator3/1
  Sum1/1 -> Sum8/2
  Rotation matrix in yaw 1/1 -> Sum3/2
  K3/1 -> Sum7/1
  Selector1/1 -> Transposed rotation matrix in yaw1/1, Transposed rotation matrix in yaw/1, Rotation matrix in yaw 1/1  "y_3=psi+psi_w"
  Gain3/1 -> Integrator4/1
  Sum8/1 -> Gain3/1
  Integrator4/1 -> nu/1, Gain6/1, Rotation matrix in yaw 1/2  "nu"
  Transposed rotation matrix in yaw1/1 -> Sum1/1
  Transposed rotation matrix in yaw/1 -> Sum8/1
  K4/1 -> Transposed rotation matrix in yaw/2
  Gain6/1 -> Sum8/3

== system ctrl_TAPM_2016/TAPM Controller w_observer/PID ==
  eta_ref : Inport
  eta : Inport  Port=2
  nu : Inport  Port=3
  Constant : Constant
  DP controller : Subsystem  AncestorBlock="marine_gnc/Control/Dynamic  Positioning /DP controller"
  DP controller1 : Subsystem  AncestorBlock="marine_gnc/Control/Dynamic  Positioning /DP controller"
  Delay : Delay  DelayLength=1  InitialCondition=0
  Integrator : Integrator  ExternalReset=rising  IgnoreLimit=on
  MATLAB Function : MATLAB Function  TreatAsAtomicUnit=on
  Multiport Switch : MultiPortSwitch  Inputs=2
  controller : S-Function  Priority=1  FunctionName=NIVeriStandIO  Parameters=width dtype portnum stime stype btype  SFunctionDeploymentMode=off  EnableBusSupport=off  mask(NI VeriStand Outport){portnum=1, width=-1, stime=-1, dtype=auto, stype=auto, btype=0}
      mask prompts: portnum "Port number:"; width "Port dimensions (-1 for dynamically sized):"; stime "Sample time (-1 for inherited):"; dtype "Data type:"; stype "Signal type:"; btype "Block type:"
      mask help: Use this outport on any level of nested subsystems to allow NI VeriStand software to map signals to it.
      mask init:
      | NIVeriStandIO_init;
      settings: CopyFcn=NIVeriStand_MDL_functions('', 'IO_copy');  DeleteFcn=NIVeriStand_MDL_functions('', 'IO_delete');  MoveFcn=set_param(gcb, 'Mask', 'on');
      mask Callback portnum: NIVeriStand_MDL_functions('', 'IO_setportnum');
      mask TypeOptions dtype: auto | double | single | int8 | uint8 | int16 | uint16 | int32 | uint32 | boolean
      mask Callback dtype: NIVeriStand_MDL_functions('', 'IO_booleansignal');
      mask TypeOptions stype: auto | real | complex
      mask Display:
      | patch([-x x], [-y y], [.90980 .81960 .32156]);
      | plot([xrad -x x xrad], [yrad -y y yrad]);
      | fprintf('NI Out%d', portnum);
  timer : S-Function  Priority=2  FunctionName=NIVeriStandIO  Parameters=width dtype portnum stime stype btype  SFunctionDeploymentMode=off  EnableBusSupport=off  mask(NI VeriStand Outport){portnum=2, width=-1, stime=-1, dtype=auto, stype=auto, btype=0}
      mask prompts: portnum "Port number:"; width "Port dimensions (-1 for dynamically sized):"; stime "Sample time (-1 for inherited):"; dtype "Data type:"; stype "Signal type:"; btype "Block type:"
      mask help: Use this outport on any level of nested subsystems to allow NI VeriStand software to map signals to it.
      mask init:
      | NIVeriStandIO_init;
      settings: CopyFcn=NIVeriStand_MDL_functions('', 'IO_copy');  DeleteFcn=NIVeriStand_MDL_functions('', 'IO_delete');  MoveFcn=set_param(gcb, 'Mask', 'on');
      mask Callback portnum: NIVeriStand_MDL_functions('', 'IO_setportnum');
      mask TypeOptions dtype: auto | double | single | int8 | uint8 | int16 | uint16 | int32 | uint32 | boolean
      mask Callback dtype: NIVeriStand_MDL_functions('', 'IO_booleansignal');
      mask TypeOptions stype: auto | real | complex
      mask Display:
      | patch([-x x], [-y y], [.90980 .81960 .32156]);
      | plot([xrad -x x xrad], [yrad -y y yrad]);
      | fprintf('NI Out%d', portnum);
  tau : Outport
  wires:
  DP controller/1(tau) -> Multiport Switch/2
  nu/1 -> DP controller1/3(nu), DP controller/3(nu)
  eta_ref/1 -> DP controller1/1(eta_ref), DP controller/1(eta_ref)
  eta/1 -> DP controller1/2(eta), MATLAB Function/3(eta), DP controller/2(eta)
  Constant/1 -> Integrator/1
  MATLAB Function/1(reset) -> Integrator/2
  Integrator/1 -> Delay/1
  MATLAB Function/2(y) -> controller/1, Multiport Switch/1
  Delay/1 -> timer/1, MATLAB Function/1(timer)
  [r_max] -> MATLAB Function/2(rmax)
  Multiport Switch/1 -> tau/1
  DP controller1/1(tau) -> Multiport Switch/3

== system ctrl_TAPM_2016/TAPM Controller w_observer/SP Generator ==
  eta : Inport
  wave_dir : Inport  Port=2
  Constant1 : Constant  Value=pi
  Gain : Gain  Gain=diag([1/(1/sqrt(90)) 1/(1/sqrt(90))])  Multiplication=Matrix(K*u)
  Gain1 : Gain  Gain=diag([1/(1/sqrt(90)) 1/(1/sqrt(90))])  Multiplication=Matrix(K*u)
  Integrator : Integrator  InitialCondition=[0 0]
  Mux : Mux  Inputs=2
  Selector : Selector  InputPortWidth=3  IndexOptions=Index vector (dialog)  Indices=[1 2]  OutputSizes=1
  Set-Point Limiter : MATLAB Function  TreatAsAtomicUnit=on
  Sum : Sum  Inputs=|++
  Sum1 : Sum  Inputs=|+-
  Transfer Fcn2 : TransferFcn  Denominator=[0.5 1]
  SP : Outport  PortDimensions=3
  wires:
  Integrator/1 -> Gain/1, Set-Point Limiter/1(sp)
  [fzp] -> Set-Point Limiter/2(fzp)
  [r_max] -> Set-Point Limiter/3(rmax)
  Mux/1 -> SP/1
  eta/1 -> Selector/1
  Transfer Fcn2/1 -> Mux/2
  Constant1/1 -> Sum/1
  Sum/1 -> Transfer Fcn2/1
  wave_dir/1 -> Sum/2
  Set-Point Limiter/1(sp_new) -> Mux/1
  Sum1/1 -> Integrator/1
  Selector/1 -> Gain1/1
  Gain/1 -> Sum1/2
  Gain1/1 -> Sum1/1

== system ctrl_TAPM_2016/Thrust allocation/Optimal angle path and constraints on rotation speed ==
  Desired Angle : Inport  Partition=on  PartitionDimension=1  PartitionWidth=1
  "initial angle " : Inport  Port=2  Partition=on  PartitionDimension=1  PartitionWidth=1
  reset : Inport  Port=3  Partition=on  PartitionDimension=1  PartitionWidth=1
  Degrees to Radians : simulink_extras/Transformations/Degrees to Radians
  Delay : Delay  DelayLength=1  InitialCondition=0
  Discrete-Time Integrator : DiscreteIntegrator  ExternalReset=either  InitialConditionSource=external  InitialConditionSetting=State (most efficient)  SampleTime=0.01  ICPrevOutput=DiscIntNeverNeededParam  ICPrevScaledInput=DiscIntNeverNeededParam
  Ensuring angle is [-pi pi] : MATLAB Function  TreatAsAtomicUnit=on
  For Each : ForEach  DisableCoverage=on  IndexMode=One-based
  MATLAB Function1 : MATLAB Function  TreatAsAtomicUnit=on
  Max Rotation Rate : Saturate  UpperLimit=Max_rotation  LowerLimit=-Max_rotation
  commanded Angle : Outport  ConcatenationDimension=1
  wires:
  Degrees to Radians/1 -> Ensuring angle is [-pi pi]/1(angle)
  Ensuring angle is [-pi pi]/1(y) -> commanded Angle/1
  Discrete-Time Integrator/1 -> Degrees to Radians/1, Delay/1  "angle"
  "initial angle "/1 -> Discrete-Time Integrator/3
  Max Rotation Rate/1 -> Discrete-Time Integrator/1
  MATLAB Function1/1(psi_D) -> Max Rotation Rate/1
  Desired Angle/1 -> MATLAB Function1/1(desired)
  reset/1 -> Discrete-Time Integrator/2
  Delay/1 -> MATLAB Function1/2(actual)

== system ctrl_TAPM_2016/Thruster control /Subsystem1 ==
  Calculated angles : Inport
  Demux : Demux  Outputs=6
  Mux : Mux  Inputs=6
  Saturation {1..6} (6 alike) : Saturate  UpperLimit=pi  LowerLimit=-pi
  Commanded angles : Outport
  wires:
  Calculated angles/1 -> Demux/1
  Demux/1 -> Saturation 1/1
  Demux/2 -> Saturation 2/1
  Demux/3 -> Saturation 3/1
  Demux/4 -> Saturation 4/1
  Demux/5 -> Saturation 5/1
  Demux/6 -> Saturation 6/1
  Mux/1 -> Commanded angles/1
  Saturation 1/1 -> Mux/1
  Saturation 6/1 -> Mux/6
  Saturation 5/1 -> Mux/5
  Saturation 2/1 -> Mux/2
  Saturation 3/1 -> Mux/3
  Saturation 4/1 -> Mux/4
